simulink model "DDS_8_channel_test"  (R2016b)
settings: Solver=VariableStepAuto  StartTime=0.0  StopTime=2^16/Fadc  RelTol=1e-3  EnableMultiTasking=on
PreLoadFcn:
  | setup
values from neighbouring files (symbols this model uses):
  Fadc = 614.4e6    (= 614400000)    [setup.m]
libraries: xbsIndex_r4 x16, CryoDetLibCMB x2, simulink x1
settings Model: Creator=Mitch  LastModifiedBy=mdewart
settings OptimizationCC: LifeSpan=inf
settings DebuggingCC: SFUnexpectedBacktrackingDiag=warning  SFNoUnconditionalDefaultTransitionDiag=warning  SFExecutionAtInitializationDiag=none
settings GRTTargetCC: TargetLangStandard=C89/C90 (ANSI)  GeneratePreprocessorConditionals=Disable all
settings ConfigComp: CovMetricSettings=dw  CovHtmlReporting=on  CovSaveCumulativeToWorkspaceVar=on  CovSaveSingleToWorkspaceVar=on  CovExternalEMLEnable=off

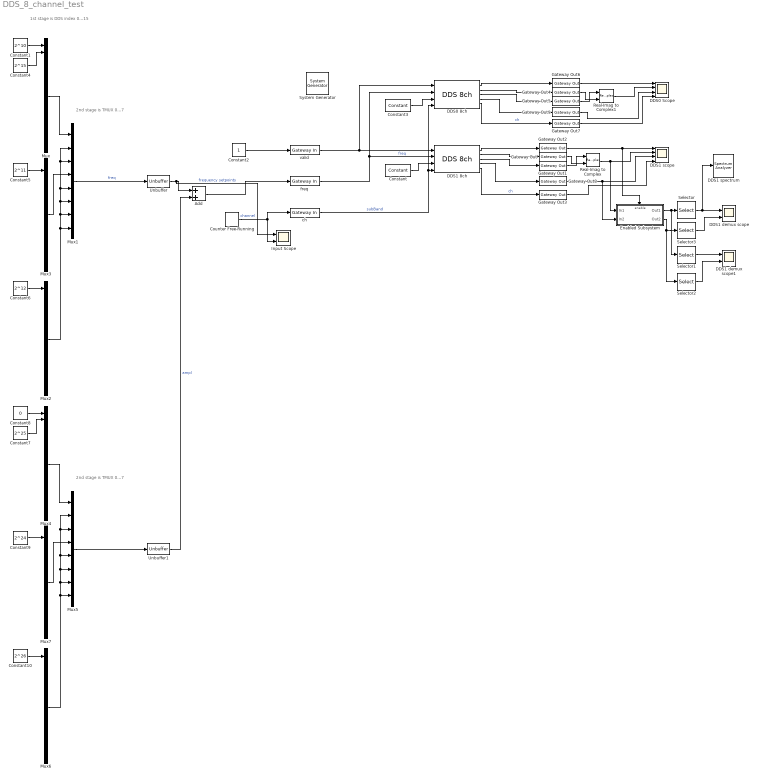
== system DDS_8_channel_test ==
  note: 2nd stage is TMUX 0...7
  note: 1st stage is DDS index 0...15
  note: 2nd stage is TMUX 0...7
  " System Generator" : xbsIndex_r4/ System Generator  Tag=genX  xilinxfamily=kintexu  part=xcku040  speed=-2-e  package=ffva1156  synthesis_tool=Vivado  clock_wrapper=Clock Enables  directory=./netlist  proj_type=Vivado  Synth_file=Vivado Synthesis Defaults  Impl_file=Vivado Implementation Defaults  testbench=off  simulink_period=2/Fadc  sysclk_period=2e9/Fadc  dcm_input_clock_period=10  incr_netlist=off  trim_vbits=Everywhere in SubSystem  dbl_ovrd=According to Block Masks  core_generation=According to Block Masks  run_coregen=off  deprecated_control=off  eval_field=0  block_type=sysgen
  Add : Sum
  Constant : xbsIndex_r4/Constant  const=1  gui_display_data_type=Fixed-point  arith_type=Unsigned  n_bits=4  bin_pt=0  preci_type=Single  exp_width=8  frac_width=24  explicit_period=off  period=1  equ=P=C  opselect=C  inp2=PCIN>>17  opr=+  inp1=P  carry=CIN  dbl_ovrd=off  block_type=constant
  Constant1 : Constant  Value=2^10  SampleTime=256/Fadc
  Constant10 : Constant  Value=2^26  SampleTime=256/Fadc
  Constant2 : Constant  SampleTime=2/Fadc
  Constant3 : xbsIndex_r4/Constant  const=0  gui_display_data_type=Fixed-point  arith_type=Unsigned  n_bits=4  bin_pt=0  preci_type=Single  exp_width=8  frac_width=24  explicit_period=off  period=1  equ=P=C  opselect=C  inp2=PCIN>>17  opr=+  inp1=P  carry=CIN  dbl_ovrd=off  block_type=constant
  Constant4 : Constant  Value=2^15  SampleTime=256/Fadc
  Constant5 : Constant  Value=2^11  SampleTime=256/Fadc
  Constant6 : Constant  Value=2^12  SampleTime=256/Fadc
  Constant7 : Constant  Value=2^25  SampleTime=256/Fadc
  Constant8 : Constant  Value=0  SampleTime=256/Fadc
  Constant9 : Constant  Value=2^24  SampleTime=256/Fadc
  Counter Free-Running : simulink/Sources/Counter Free-Running  NumBits=7  tsamp=2/Fadc
  DDS0 8ch : CryoDetLibCMB/DDS 8ch
  DDS0 Scope : Scope  NumInputPorts=4
  DDS1 8ch : CryoDetLibCMB/DDS 8ch
  DDS1 demux scope : Scope  NumInputPorts=2
  DDS1 demux scope1 : Scope  NumInputPorts=2
  DDS1 scope : Scope  NumInputPorts=4
  DDS1 spectrum : SpectrumAnalyzer
  Enabled Subsystem : Subsystem  TreatAsAtomicUnit=on
  Gateway Out{,1..9} (10 alike) : xbsIndex_r4/Gateway Out  inherit_from_input=off  hdl_port=on  rows=1  columns=1  UseAsDAC=off  DACChannel='1'  interface=None  automatic_assignment=on  address_offset=hex2dec('00')  intf_name=''  intf_description=''  timing_constraint=None  locs_specified=off  LOCs={}  io_standard={}  block_type=gatewayout
  Input Scope : Scope  NumInputPorts=2
  Mux{,2..4,6..7} (6 alike) : Mux  Inputs=16
  Mux1 : Mux  Inputs=8
  Mux5 : Mux  Inputs=8
  Real-Imag to Complex : RealImagToComplex
  Real-Imag to Complex1 : RealImagToComplex
  Selector : Selector  InputPortWidth=8  IndexOptions=Index vector (dialog)  Indices=[0+1]  OutputSizes=1
  Selector1 : Selector  InputPortWidth=8  IndexOptions=Index vector (dialog)  Indices=[3+1]  OutputSizes=1
  Selector2 : Selector  InputPortWidth=8  IndexOptions=Index vector (dialog)  Indices=[3+1]  OutputSizes=1
  Selector3 : Selector  InputPortWidth=8  IndexOptions=Index vector (dialog)  Indices=[0+1]  OutputSizes=1
  Unbuffer : Unbuffer  SampleBasedProcessing=Same as frame based
  Unbuffer1 : Unbuffer  SampleBasedProcessing=Same as frame based
  ch : xbsIndex_r4/Gateway In  gui_display_data_type=Fixed-point  arith_type=Unsigned  n_bits=7  bin_pt=0  preci_type=Single  exp_width=8  frac_width=24  rows=1  columns=1  quantization="Round  (unbiased: +/- Inf)"  overflow=Saturate  period=2/Fadc  UseAsADC=off  ADCChannel='1'  interface=None  automatic_assignment=on  address_offset=hex2dec('00')  intf_name=''  intf_description=''  default_value=0  timing_constraint=None  locs_specified=off  LOCs={}  io_standard={}  inherit_from_input=off  hdl_port=on  dbl_ovrd=off  block_type=gatewayin
  freq : xbsIndex_r4/Gateway In  gui_display_data_type=Fixed-point  arith_type=Unsigned  n_bits=32  bin_pt=0  preci_type=Single  exp_width=8  frac_width=24  rows=1  columns=1  quantization="Round  (unbiased: +/- Inf)"  overflow=Saturate  period=2/Fadc  UseAsADC=off  ADCChannel='1'  interface=None  automatic_assignment=on  address_offset=hex2dec('00')  intf_name=''  intf_description=''  default_value=0  timing_constraint=None  locs_specified=off  LOCs={}  io_standard={}  inherit_from_input=off  hdl_port=on  dbl_ovrd=off  block_type=gatewayin
  valid : xbsIndex_r4/Gateway In  gui_display_data_type=Boolean  arith_type=Boolean  n_bits=1  bin_pt=0  preci_type=Single  exp_width=8  frac_width=24  rows=1  columns=1  quantization="Round  (unbiased: +/- Inf)"  overflow=Saturate  period=2/Fadc  UseAsADC=off  ADCChannel='1'  interface=None  automatic_assignment=on  address_offset=hex2dec('00')  intf_name=''  intf_description=''  default_value=0  timing_constraint=None  locs_specified=off  LOCs={}  io_standard={}  inherit_from_input=off  hdl_port=on  dbl_ovrd=off  block_type=gatewayin
  wires:
  Real-Imag to Complex/1 -> Enabled Subsystem/1(In1), DDS1 scope/2
  Constant2/1 -> valid/1
  Gateway Out2/1 -> DDS1 scope/1, Enabled Subsystem/Enable
  Counter Free-Running/1 -> Input Scope/2, ch/1  "channel"
  Real-Imag to Complex1/1 -> DDS0 Scope/2
  Gateway Out6/1 -> DDS0 Scope/1
  freq/1 -> DDS1 8ch/2, DDS0 8ch/2  "freq"
  Mux1/1 -> Unbuffer/1  "freq"
  Mux/1 -> Mux1/1
  Constant4/1 -> Mux/2
  Mux2/1 -> Mux1/7, Mux1/6, Mux1/5, Mux1/3, Mux1/2, Mux1/8
  Enabled Subsystem/1(Out1) -> Selector1/1, Selector/1
  Selector/1 -> DDS1 demux scope/1, DDS1 spectrum/1
  Constant1/1 -> Mux/1
  Mux3/1 -> Mux1/4
  Constant5/1 -> Mux3/2
  Constant6/1 -> Mux2/1
  Constant/1 -> DDS1 8ch/3
  Constant3/1 -> DDS0 8ch/3
  valid/1 -> DDS1 8ch/1, DDS0 8ch/1
  ch/1 -> DDS1 8ch/4, DDS0 8ch/4  "subBand"
  DDS1 8ch/1 -> Gateway Out2/1
  DDS1 8ch/2 -> Gateway Out/1
  DDS1 8ch/3 -> Gateway Out1/1
  Gateway Out1/1 -> Real-Imag to Complex/1
  Gateway Out/1 -> Real-Imag to Complex/2
  Gateway Out5/1 -> Real-Imag to Complex1/1
  Gateway Out4/1 -> Real-Imag to Complex1/2
  DDS0 8ch/1 -> Gateway Out6/1
  DDS0 8ch/2 -> Gateway Out4/1
  DDS0 8ch/3 -> Gateway Out5/1
  DDS1 8ch/5 -> Gateway Out3/1  "ch"
  DDS0 8ch/5 -> Gateway Out7/1  "ch"
  Mux5/1 -> Unbuffer1/1
  Mux4/1 -> Mux5/1
  Mux6/1 -> Mux5/8, Mux5/2, Mux5/3, Mux5/5, Mux5/6, Mux5/7
  Mux7/1 -> Mux5/4
  Constant9/1 -> Mux7/2
  Constant10/1 -> Mux6/1
  Gateway Out7/1 -> DDS0 Scope/4
  Gateway Out9/1 -> DDS0 Scope/3
  DDS0 8ch/4 -> Gateway Out9/1
  DDS1 8ch/4 -> Gateway Out8/1
  Gateway Out3/1 -> DDS1 scope/4
  Gateway Out8/1 -> Enabled Subsystem/2(In2), DDS1 scope/3
  Enabled Subsystem/2(Out2) -> Selector3/1, Selector2/1
  Selector3/1 -> DDS1 demux scope/2
  Selector1/1 -> DDS1 demux scope1/1
  Selector2/1 -> DDS1 demux scope1/2
  Constant7/1 -> Mux4/2
  Constant8/1 -> Mux4/1
  Unbuffer/1 -> Input Scope/1, Add/1  "frequency setpoints"
  Add/1 -> freq/1
  Unbuffer1/1 -> Add/2  "ampl"

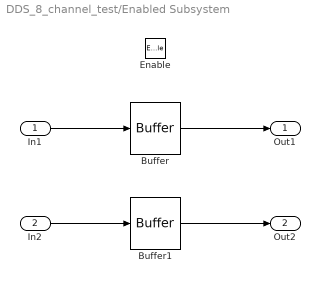
== system DDS_8_channel_test/Enabled Subsystem ==
  In1 : Inport
  In2 : Inport  Port=2
  Enable : EnablePort
  Buffer : Buffer  N=8  TreatMby1Signals=One channel  OutputFrames=off
  Buffer1 : Buffer  N=8  TreatMby1Signals=One channel  OutputFrames=off
  Out1 : Outport
  Out2 : Outport  Port=2
  wires:
  In1/1 -> Buffer/1
  Buffer/1 -> Out1/1
  In2/1 -> Buffer1/1
  Buffer1/1 -> Out2/1
